simulink model "simulink_model"  (R2025a)
settings: Solver=ode45  StartTime=0.0  StopTime=Inf  FixedStep=.01  RelTol=1e-3  EnableMultiTasking=on
values from neighbouring files (symbols this model uses):
  A = [-1.064, 1.000; 290.26, 0.00]    [missile_gnc.m]
  B = [-0.25; -331.40]    [missile_gnc.m]
  C = [-123.34, 0.00; 0.00, 1.00]    [missile_gnc.m]
  D = [-13.41; 0.00]    [missile_gnc.m]
  dT1 = 0.75    [missile_gnc.m]
  dT2 = 0.25    [missile_gnc.m]
  ELEV_INIT = 10000    [missile_gnc.m]
  ELEV_TARGET = 795    [missile_gnc.m]
  LAT_INIT = 34.2329    [missile_gnc.m]
  LAT_OBS = 34.61916    [missile_gnc.m]
  LAT_TARGET = 34.6588    [missile_gnc.m]
  LON_INIT = -119.4573    [missile_gnc.m]
  LON_OBS = -118.8429    [missile_gnc.m]
  LON_TARGET = -118.769745    [missile_gnc.m]
undefined symbols (not defined in the file or in its folder): K, L
libraries: simulink x3, slpidlib x1, aerolibanimutils x1
settings Model: Creator=vinay  LastModifiedBy=naitik
settings SolverCC: AlgebraicLoopSolver=TrustRegion
settings DataIOCC: LimitDataPoints=on  SaveFormat=Array  ReturnWorkspaceOutputs=off
settings OptimizationCC: LifeSpan=inf
settings DebuggingCC: UnconnectedInputMsg=warning  UnconnectedOutputMsg=warning  UnconnectedLineMsg=warning  SFUnexpectedBacktrackingDiag=warning  SFNoUnconditionalDefaultTransitionDiag=warning  SFExecutionAtInitializationDiag=none  ArithmeticOperatorsInVariantConditions=warning
settings HardwareCC: ProdBitPerPointer=32.0  ProdBitPerSizeT=32.0  ProdBitPerPtrDiffT=32.0  ProdLargestAtomicFloat=None  ProdIntDivRoundTo=Undefined  ProdEndianess=Unspecified  ProdWordSize=32.0  ProdHWDeviceType=32-bit Generic
settings ModelReferenceCC: PropagateSignalLabelsOutOfModel=off
settings SFSimCC: SimUseLocalCustomCode=off  CustomCodeUndefinedFunction=UseInterfaceOnly
settings RTWCC: RTWUseLocalCustomCode=off  GPUComputeCapability=3.5
settings CodeAppCC: StateflowObjectComments=on
settings GRTTargetCC: TargetLangStandard=C89/C90 (ANSI)
settings ConfigComp: CovMetricSettings=dw  CovSaveCumulativeToWorkspaceVar=on  CovSaveSingleToWorkspaceVar=on  CovExternalEMLEnable=off

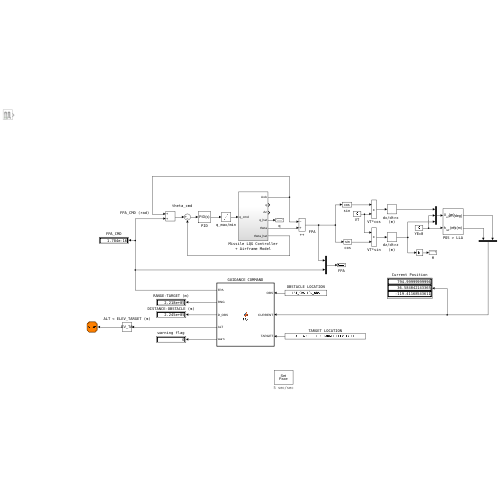
[thumbnail: Simulink's stored preview of the top-level diagram]
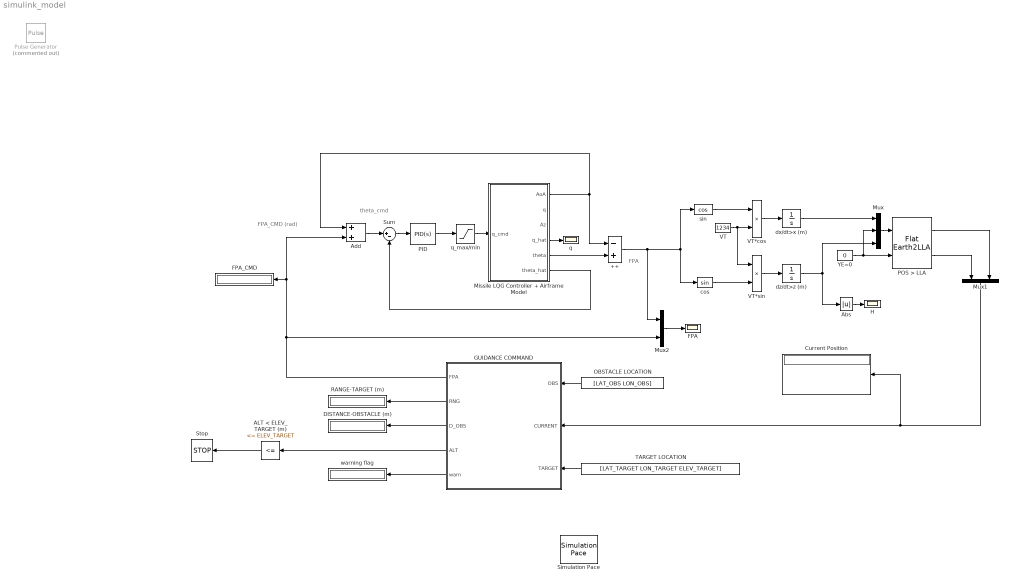
== system simulink_model ==
  note: FPA_CMD (rad)
  note: theta_cmd
  note: FPA
  ++ : Sum  Inputs=-+
  ALT < ELEV_TARGET (m) : simulink/Logic and Bit Operations/Compare To Constant  relop=<=  const=ELEV_TARGET  OutDataTypeStr=boolean
  Abs : Abs  SaturateOnIntegerOverflow=off
  Add : Sum
  Current Position : Display
  DISTANCE-OBSTACLE (m) : Display
  FPA : Scope
      settings: TimeSpan=80  ActiveDisplayYMinimum=-0.01  ActiveDisplayYMaximum=0.13  DataLoggingVariableName=ScopeData4  DataLoggingSaveFormat=Array
  FPA_CMD : Display
  GUIDANCE COMMAND : MATLAB Function  TreatAsAtomicUnit=on
  H : Scope
      settings: TimeSpan=80  ActiveDisplayYMinimum=-0.01  ActiveDisplayYMaximum=0.13  DataLoggingVariableName=ScopeData2  DataLoggingSaveFormat=Array
  Missile LQG Controller + Airframe Model : Subsystem
  Mux : Mux  Inputs=3
  Mux1 : Mux  Inputs=2
  Mux2 : Mux  Inputs=2
  OBSTACLE LOCATION : Constant  Value=[LAT_OBS LON_OBS]
  PID : slpidlib/PID Controller  Controller=PID  Form=Parallel  TimeDomain=Continuous-time  UseExternalTs=off  SampleTime=-1  IntegratorMethod=Forward Euler  FilterMethod=Forward Euler  ControllerParametersSource=internal  P=-1.0  I=0  UseKiTs=off  D=0  UseExternalDerivativeSource=off  N=100  UseFilter=on  TunerSelectOption=Transfer Function Based (PID Tuner App)  InitialConditionSource=internal  InitialConditionForIntegrator=0  InitialConditionForFilter=0  DifferentiatorICPrevScaledInput=0  ExternalReset=none  TrackingMode=off  Kt=1  LimitOutput=off  SatLimitsSource=internal  UpperSaturationLimit=inf  LowerSaturationLimit=-inf  LinearizeAsGain=on  AntiWindupMode=none  Kb=1  LimitIntegrator=off  UpperIntegratorSaturationLimit=inf  LowerIntegratorSaturationLimit=-inf  POutMin=[]  POutMax=[]  IOutMin=[]  IOutMax=[]  DOutMin=[]  DOutMax=[]  NOutMin=[]  NOutMax=[]  SumOutMin=[]  SumOutMax=[]  SaturationOutMin=[]  SaturationOutMax=[]  PParamMin=[]  PParamMax=[]  IParamMin=[]  IParamMax=[]  DParamMin=[]  DParamMax=[]  NParamMin=[]  NParamMax=[]  KbParamMin=[]  KbParamMax=[]  KtParamMin=[]  KtParamMax=[]  KbOutMin=[]  KbOutMax=[]  KtOutMin=[]  KtOutMax=[]  IntegratorOutMin=[]  IntegratorOutMax=[]  FilterOutMin=[]  FilterOutMax=[]  SumI1OutMin=[]  SumI1OutMax=[]  SumI2OutMin=[]  SumI2OutMax=[]  SumI3OutMin=[]  SumI3OutMax=[]  SumI4OutMin=[]  SumI4OutMax=[]  SumDOutMin=[]  SumDOutMax=[]  DifferentiatorOutMin=[]  DifferentiatorOutMax=[]  FilterDiffOutCoefMin=[]  FilterDiffOutCoefMax=[]  ReciprocalOutMin=[]  ReciprocalOutMax=[]  SumDenOutMin=[]  SumDenOutMax=[]  SumNumOutMin=[]  SumNumOutMax=[]  DivideOutMin=[]  DivideOutMax=[]  UdiffTsProdOutMin=[]  UdiffTsProdOutMax=[]  NTsProdOutMin=[]  NTsProdOutMax=[]  UintegralTsProdOutMin=[]  UintegralTsProdOutMax=[]  UngainTsProdOutMin=[]  UngainTsProdOutMax=[]  ClampingZeroOutDataTypeStr=Inherit: Inherit via back propagation  ClampingZeroOutMin=[]  ClampingZeroOutMax=[]  FilterDenConstantOutDataTypeStr=Inherit: Inherit via back propagation  FilterDenConstantOutMin=[]  FilterDenConstantOutMax=[]  PCopyOutDataTypeStr=Inherit: Inherit via back propagation  PCopyOutMin=[]  PCopyOutMax=[]  NCopyOutDataTypeStr=Inherit: Inherit via back propagation  NCopyOutMin=[]  NCopyOutMax=[]  IntegratorContinuousStateAttributes=''  IntegratorStateMustResolveToSignalObject=off  IntegratorRTWStateStorageClass=Auto  FilterContinuousStateAttributes=''  FilterStateMustResolveToSignalObject=off  FilterRTWStateStorageClass=Auto  ParallelPVariant=InternalParameters  IdealPVariant=Disabled  IVariant=InternalParameters  DVariant=InternalParameters  IntegratorVariant=Discrete  SatVariant=Disabled  AWVariant=Passthrough  PCopyVariant=Disabled  TRVariant=Disabled  FdbkBlocksVariant=Forward  IdealPFdbkVariant=Disabled  SatFdbkVariant=Disabled  DerivativeFilterVariant=ForwardEulerFilter  NVariant=InternalParameters  NCopyVariant=Disabled  FilterICVariant=InternalICsFilter  IntegratorICVariant=InternalICs  ExternalResetVariant=Disabled  TRSumVariant=Passthrough  SumFdbkVariant=Disabled  SumVariant=Sum_PID  TsampFilterVariant=InternalTs  TsampNgainVariant=Passthrough  TsampIntegralVariant=Disabled_SignalSpec  ExternalSaturationOutDataTypeStr=Inherit: Same as second input  DerivativeSourceVariant=ErrorSignal  PreIntVariant=InternalPreInt
  POS > LLA : FlatEarth2LLA  R=6378137  LL0=[LAT_INIT LON_INIT]  psi=yaw_init
  Pulse Generator : DiscretePulseGenerator  Commented=on  PulseType=Time based  Amplitude=0.75  Period=60  PulseWidth=50
  RANGE-TARGET (m) : Display
  Simulation Pace : aerolibanimutils/Simulation Pace  SimulationPace=5  SleepMode=MATLAB Thread  OutputPaceError=off  SampleTime=1/30
      settings: AttributesFormatString=%<SimulationPace> sec/sec
  Stop : Stop
  Sum : Sum  Inputs=|+-
  TARGET LOCATION : Constant  Value=[LAT_TARGET LON_TARGET ELEV_TARGET]
  VT : Constant  Value=1234
  VT*cos : Product
  VT*sin : Product
  YE=0 : Constant  Value=0
  cos : Trigonometry
  dx/dt>x (m) : Integrator
  dz/dt>z (m) : Integrator  InitialCondition=-ELEV_INIT
  q : Scope
      settings: TimeSpan=78  DataLoggingSaveFormat=Array
  q_max/min : Saturate
  sin : Trigonometry  Operator=cos
  warning flag : Display
  wires:
  Sum/1 -> PID/1
  Missile LQG Controller + Airframe Model/6(theta_hat) -> Sum/2
  PID/1 -> q_max/min/1
  q_max/min/1 -> Missile LQG Controller + Airframe Model/1(q_cmd)
  GUIDANCE COMMAND/1(FPA) -> Mux2/2, FPA_CMD/1, Add/2
  Missile LQG Controller + Airframe Model/1(AoA) -> Add/1, ++/1
  Add/1 -> Sum/1
  Missile LQG Controller + Airframe Model/5(theta) -> ++/2
  VT/1 -> VT*cos/2, VT*sin/1
  sin/1 -> VT*cos/1
  ++/1 -> Mux2/1, cos/1, sin/1
  cos/1 -> VT*sin/2
  VT*sin/1 -> dz/dt>z (m)/1
  VT*cos/1 -> dx/dt>x (m)/1
  YE=0/1 -> Mux/2, POS > LLA/2
  Mux/1 -> POS > LLA/1
  dz/dt>z (m)/1 -> Mux/3, Abs/1
  dx/dt>x (m)/1 -> Mux/1
  OBSTACLE LOCATION/1 -> GUIDANCE COMMAND/1(OBS)
  TARGET LOCATION/1 -> GUIDANCE COMMAND/3(TARGET)
  POS > LLA/2 -> Mux1/1
  POS > LLA/1 -> Mux1/2
  Mux1/1 -> Current Position/1, GUIDANCE COMMAND/2(CURRENT)
  GUIDANCE COMMAND/2(RNG) -> RANGE-TARGET (m)/1
  GUIDANCE COMMAND/4(ALT) -> ALT < ELEV_TARGET (m)/1
  ALT < ELEV_TARGET (m)/1 -> Stop/1
  Missile LQG Controller + Airframe Model/4(q_hat) -> q/1
  Mux2/1 -> FPA/1
  GUIDANCE COMMAND/3(D_OBS) -> DISTANCE-OBSTACLE (m)/1
  GUIDANCE COMMAND/5(warn) -> warning flag/1
  Abs/1 -> H/1

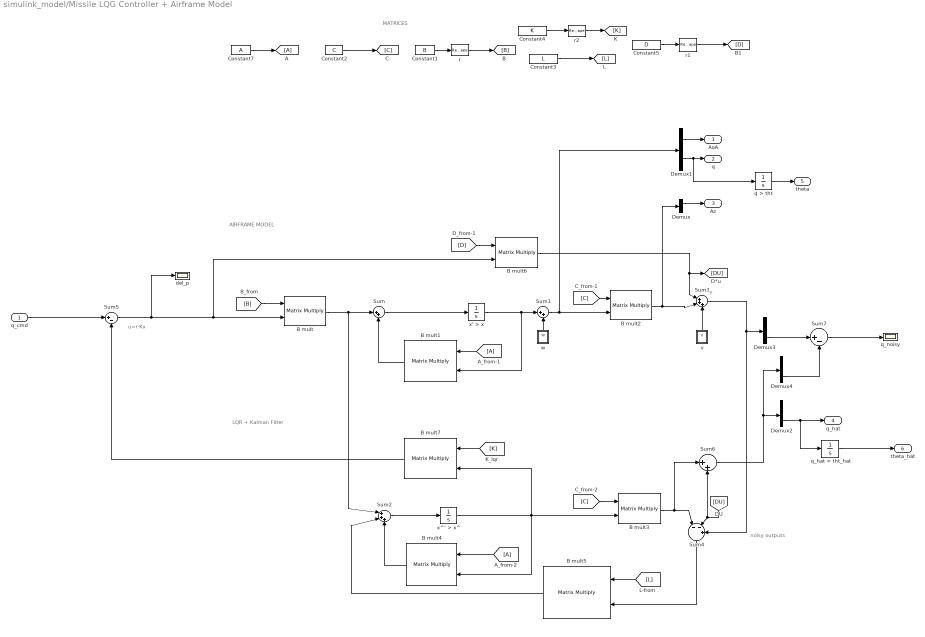
== system simulink_model/Missile LQG Controller + Airframe Model ==
  note: noisy
      | outputs
  note: LQR + Kalman Filter
  note: AIRFRAME MODEL
  note: u=r-Kx
  note: Y
  note: MATRICES
  q_cmd : Inport
  A : Goto
  A_from-1 : From
  A_from-2 : From
  B mult{,1..7} (8 alike) : Product  Multiplication=Matrix(*)  RndMeth=Zero
  Constant1 : Constant  Value=B
  Constant2 : Constant  Value=C
  Constant3 : Constant  Value=L
  Constant4 : Constant  Value=K
  Constant5 : Constant  Value=D
  Constant7 : Constant  Value=A
  Demux{,1..4} (5 alike) : Demux  Outputs=2
  Sum : Sum  Inputs=|++
  Sum1 : Sum  Inputs=|++
  Sum2 : Sum  Inputs=|+++
  Sum3 : Sum  Inputs=|+++
  Sum4 : Sum  Inputs=|--+
  Sum5 : Sum  Inputs=|+-
  Sum6 : Sum  Inputs=|++
  Sum7 : Sum  Inputs=|+-
  del_p : Scope
      settings: TimeSpan=78  DataLoggingSaveFormat=Array
  q > tht : Integrator
  q_hat > tht_hat : Integrator
  q_noisy : Scope
      settings: TimeSpan=78  DataLoggingVariableName=ScopeData3  DataLoggingSaveFormat=Array
  r : Reshape  OutputDimensionality=Customize  OutputDimensions=[2,1]
  r1 : Reshape  OutputDimensionality=Customize  OutputDimensions=[2,1]
  r2 : Reshape  OutputDimensionality=Customize  OutputDimensions=[1,2]
  v : Subsystem
  w : Subsystem
  x' > x : Integrator
  x^' > x^ : Integrator  InitialCondition=[0.01;0.01]
  AoA : Outport
  q : Outport  Port=2
  Az : Outport  Port=3
  q_hat : Outport  Port=4
  theta : Outport  Port=5
  theta_hat : Outport  Port=6
  wires:
  B mult2/1 -> Demux/1, Sum3/2
  [D] -> B mult6/1
  v/1(v) -> Sum3/3
  [B] -> B mult/1
  B mult6/1 -> [DU], Sum3/1
  Sum/1 -> x' > x/1
  B mult3/1 -> Sum6/1, Sum4/1
  A_from-1/1 -> B mult1/1
  Sum1/1 -> Demux1/1, B mult2/2
  [C] -> B mult3/1
  Sum4/1 -> B mult5/2
  x' > x/1 -> B mult1/2, Sum1/1
  A_from-2/1 -> B mult4/1
  Sum2/1 -> x^' > x^/1
  B mult4/1 -> Sum2/3
  B mult/1 -> Sum/1, Sum2/1
  B mult1/1 -> Sum/2
  [C] -> B mult2/1
  B mult5/1 -> Sum2/2
  [K] -> B mult7/1
  w/1(w) -> Sum1/2
  [DU] -> Sum6/2, Sum4/2
  B mult7/1 -> Sum5/2
  Sum5/1 -> del_p/1, B mult6/2, B mult/2
  Demux/1 -> Az/1
  Demux1/1 -> AoA/1
  Demux1/2 -> q > tht/1, q/1
  Demux2/2 -> q_hat > tht_hat/1, q_hat/1
  Constant7/1 -> A/1
  Constant1/1 -> r/1
  Constant2/1 -> [C]
  Constant3/1 -> [L]
  Constant4/1 -> r2/1
  r/1 -> [B]
  r1/1 -> [D]
  Constant5/1 -> r1/1
  r2/1 -> [K]
  q_hat > tht_hat/1 -> theta_hat/1
  q > tht/1 -> theta/1
  Sum6/1 -> Demux2/1, Demux4/1
  q_cmd/1 -> Sum5/1
  Sum7/1 -> q_noisy/1
  Sum3/1 -> Demux3/1, Sum4/3
  Demux3/2 -> Sum7/1
  Demux4/2 -> Sum7/2
  x^' > x^/1 -> B mult4/2, B mult7/2, B mult3/2
  [L] -> B mult5/1

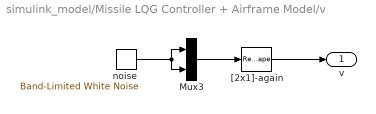
== system simulink_model/Missile LQG Controller + Airframe Model/v ==
  Mux3 : Mux  Inputs=2
  "[2x1]-again" : Reshape  OutputDimensionality=Customize  OutputDimensions=[2,1]
  noise : simulink/Sources/Band-Limited White Noise  Cov=[0.00001]  Ts=dT2  seed=[23341]
  v : Outport
  wires:
  "[2x1]-again"/1 -> v/1
  noise/1 -> Mux3/2, Mux3/1
  Mux3/1 -> "[2x1]-again"/1

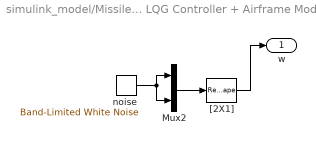
== system simulink_model/Missile LQG Controller + Airframe Model/w ==
  Mux2 : Mux  Inputs=2
  "[2X1]" : Reshape  OutputDimensionality=Customize  OutputDimensions=[2,1]
  noise : simulink/Sources/Band-Limited White Noise  Cov=0.00000001  Ts=dT1  seed=[23341]
  w : Outport
  wires:
  Mux2/1 -> "[2X1]"/1
  "[2X1]"/1 -> w/1
  noise/1 -> Mux2/1, Mux2/2

== matlab function simulink_model/GUIDANCE COMMAND ==
  data: OBS input; FPA output; CURRENT input; TARGET input; RNG output; D_OBS output; ALT output; warn output
function [FPA,RNG,D_OBS,ALT,warn]= FPA(OBS, CURRENT, TARGET)
%#codegen

R = 6371e3; %earth radius (m)
d2r = pi/180;

%OBSTACLE LOCATION
LAT_OBS = OBS(1);
LON_OBS = OBS(2);

%OBSTACLE THRESHOLD (m)
thres = 2000;

%TARGET location
LAT_TARGET = TARGET(1);
LON_TARGET = TARGET(2);
ELEV_TARGET = TARGET(3); %m - MSL

%CURRENT location
LAT_CUR = CURRENT(2);
LON_CUR = CURRENT(3);
ELEV_CUR = CURRENT(1);

%% distance remaining to target----------------------------------

l1 = LAT_CUR*d2r;
u1 = LON_CUR*d2r;
l2 = LAT_TARGET*d2r;
u2 = LON_TARGET*d2r;
dh = abs(ELEV_TARGET-ELEV_CUR);

dl = l2-l1;
du = u2-u1;

a = sin(dl/2)^2 + cos(l1)*cos(l2)*sin(du/2)^2;
c = 2*atan2(sqrt(a),sqrt(1-a));
d = R*c; %horizontal distance (in m)

%% distance from the obstacle----------------------------------

l3 = LAT_OBS*d2r;
u3 = LON_OBS*d2r;

dl = l3-l1;
du = u3-u1;

a = sin(dl/2)^2 + cos(l1)*cos(l2)*sin(du/2)^2;
c = 2*atan2(sqrt(a),sqrt(1-a));
d_obs = R*c; %horizontal distance (in m)


%% current range (from target) - range > distance
range = sqrt(d^2+dh^2);

%% calculate commanded flight path setpoint - based on d_obs and range

if abs(d_obs)>=thres
    w = 0;
    FPA_CMD = atan(dh/d); %rad
else
    %when <2000m, trigger warning
    w = 1;
    FPA_CMD = 0;
end

%% set output variables

FPA = FPA_CMD;

RNG = range;

D_OBS = d_obs;

warn = w;

ALT = ELEV_CUR;
